simulink model "CLNN_sim_3dof_2NN"  (R2024b)
settings: Solver=ode1  StartTime=0.0  StopTime=T_all  FixedStep=T_sample  RelTol=1e-3
values from neighbouring files (symbols this model uses):
  a1 = m1 * lc1^2 + I1 + (m2 + m3) * l1^2    [plant_robot_3DoF_2NN.m]    (also in setting_3dof_2NN.m = 8.9995)
  a2 = I2 + m2 * lc2^2 + m3 * l2^2    [plant_robot_3DoF_2NN.m]    (also in setting_3dof_2NN.m = 8.9989)
  cl_tf = 300    [run_CLNN_3dof_2NN.m]
  cl_tf1 = 0    [run_CLNN_3dof_2NN.m]
  cl_tf2 = 1050    [run_CLNN_3dof_2NN.m]
  hidden_neure_count_q = 50    [run_CLNN_3dof_2NN.m]
  hidden_neure_count_s = 30    [run_CLNN_3dof_2NN.m]
  kq1 = 0.0026    [setting_3dof_2NN.m]
  kq2 = 0.0011    [setting_3dof_2NN.m]
  lamda = 5    [run_CLNN_3dof_2NN.m]
  lamda_cl = 0.2    [run_CLNN_3dof_2NN.m]
  lamda_cl_s = 0.2    [run_CLNN_3dof_2NN.m]
  learn_time = 100    [run_CLNN_3dof_2NN.m]
  M = [0.001 0 0 ... (first row only)    [run_CLNN_3dof_2NN.m]
  N = 3    [setting_3dof_2NN.m]
  noise_cov = 0    [setting_3dof_2NN.m]
  output_dimension_q = 1*N    [run_CLNN_3dof_2NN.m]
  output_dimension_s = 1*N    [run_CLNN_3dof_2NN.m]
  qd20 = 0    [run_CLNN_3dof_2NN.m]
  use_Tqr = 0    [run_CLNN_3dof_2NN.m]
(part 2 of 2)

== matlab function CLNN_sim_3dof_2NN/s/sd1 ==
  data: t input; q output; q2 output; dq2 output; dqq2 output; dqqq2 output; dqqqq2 output; learn_time input
function [q,q2,dq2,dqq2,dqqq2,dqqqq2]  = fcn(t, learn_time)

%% sim s1

a  = 0;  %paper pi / 12
w = 0;   %paper 2

a1 = 0.8 * pi / 1; %paper 0.8 * pi / 1
w1 = pi / 6;        % paper pi / 6  

if t> learn_time
    a1 = 0.8 * pi / 1; %paper 0.8 * pi / 1
    w1 = pi / 4;        % paper pi / 6  
end

q = 16 *( a1 * sin(w1 * t) + 1* 8 * pi);  %paper 1* 3 * pi


q2 = a * cos(w * t) - a + a1 * sin(w1 * t);
dq2 = -a * w * sin(w * t) + a1 * w1 * cos(w1 * t);
dqq2 = -a * w * w * cos(w * t) - a1 * w1 * w1 * sin(w1 * t);
dqqq2 = 0;
dqqqq2 = 0;
return;

== matlab function CLNN_sim_3dof_2NN/s/sd2 ==
  data: t input; q output; q2 output; dq2 output; dqq2 output; dqqq2 output; dqqqq2 output; learn_time input
function [q,q2,dq2,dqq2,dqqq2,dqqqq2]  = fcn(t, learn_time)
%% sim s2
a  = 0;  %paper pi / 12
w = 0;   %paper 2

a1 = 0.2 * pi / 1; % paper 0.2 * pi / 1; 
w1 = pi / 5;   % paper pi /5   

% if t > 80
%     w1 = pi / 8;
% elseif t > 50
%      w1 = pi / 7;
% elseif t > 20
%      w1 = pi / 6;
% end

if t> learn_time
    a1 = 0.2 * pi / 1; %paper 0.8 * pi / 1
    w1 = pi / 4;        % paper pi / 6  
end

q = 16 *( a1 * sin(w1 * t) + 1* 6 * pi);   % paper 1*3 * pi

q2 = a * cos(w * t) - a + a1 * sin(w1 * t) + pi/2;
dq2 = -a * w * sin(w * t) + a1 * w1 * cos(w1 * t);
dqq2 = -a * w * w * cos(w * t) - a1 * w1 * w1 * sin(w1 * t);
dqqq2 = 0;
dqqqq2 = 0;
return;

== matlab function CLNN_sim_3dof_2NN/s/sd3 ==
  data: t input; q output; q2 output; dq2 output; dqq2 output; dqqq2 output; dqqqq2 output; learn_time input
function [q,q2,dq2,dqq2,dqqq2,dqqqq2]  = fcn(t, learn_time)
%% sim s3
a  = 0;  %paper pi / 12
w = 0;   %paper 2
a1 = 0.2 * pi / 1; % paper 0.2 * pi / 1; 
w1 = pi / 5;   % paper pi /5   

if t> learn_time
    a1 = 0.2 * pi / 1; %paper 0.8 * pi / 1
    w1 = pi / 4;        % paper pi / 6  
end

q = 16 *( a1 * sin(w1 * t) + 1* 1* pi);   % paper 1*3 * pi

q2 = a * cos(w * t) - a + a1 * sin(w1 * t);
dq2 = -a * w * sin(w * t) + a1 * w1 * cos(w1 * t);
dqq2 = -a * w * w * cos(w * t) - a1 * w1 * w1 * sin(w1 * t);
dqqq2 = 0;
dqqqq2 = 0;
return;

== matlab function CLNN_sim_3dof_2NN/Theta_q/MATLAB Function Theta ==
  data: phi_filter_q input; phi_filter_phi_filter_q output; hidden_neure_count_q input
function phi_filter_phi_filter_q  = fcn(phi_filter_q,hidden_neure_count_q)
phi_filter_phi_filter_m = phi_filter_q * phi_filter_q';

phi_filter_phi_filter_q = phi_filter_phi_filter_m;
% phi_filter_phi_filter = zeros(625,625);

== matlab function CLNN_sim_3dof_2NN/THeta_WW_q/MATLAB Function Theta_W ==
  data: phi_filter_q input; phi_filter_W_q output; w_un_q_filter input; w_un_s_filter input
function phi_filter_W_q  = fcn(phi_filter_q,  w_un_q_filter, w_un_s_filter)
% w_un_filter = [w_un_q_filter; w_un_s_filter];
phi_filter_W_q = phi_filter_q * w_un_q_filter';

== matlab function CLNN_sim_3dof_2NN/THeta_WW_q/MATLAB Function ==
  data: u input; y output; t input; cl_tf1 input; cl_tf2 input
function y = fcn(u,t,cl_tf1, cl_tf2)
if t>cl_tf1 && t< cl_tf2
    y = u;
else
    y = zeros(51,3);  %41 x 6   (61,2)
end

== matlab function CLNN_sim_3dof_2NN/MATLAB Function6 ==
  data: output input; w_un_hat output; epsion output; w_norm_q output; w_norm_s output; controlu1 output; controlu2 output; u_theta1 output; u_theta2 output; pd_u output; model_u output; W_q output; hidden_neure_count_q input; hidden_neure_count_s input; N input; q input; W_s output
function [w_un_hat, epsion, w_norm_q,w_norm_s,controlu1, controlu2, u_theta1, u_theta2,pd_u, model_u, W_q, W_s] = fcn(output, hidden_neure_count_q,hidden_neure_count_s,N,q)
N = 3;
output_dimension = 2*N;

w_un_hat = output(1:output_dimension);
epsion =  output((output_dimension + 1):(2 * output_dimension));
controlu1 = output((2 * output_dimension +1):(2 * output_dimension + N));
controlu2 = output((2 * output_dimension + N +1):(2 * output_dimension + 2 * N));

pd_u = 0;
model_u = 0;
u_theta1 = q - controlu1;
u_theta2 = q - controlu2;


hidden_neure_count_q = 50; %40
hidden_neure_count_s = 30;
N_wq = N *(hidden_neure_count_q +1);
N_ws = N *(hidden_neure_count_s +1);

w_norm_temp_q = 0;
for i = (2 * output_dimension + 2 * N + 1):(N_wq + 2 * output_dimension + 2 * N)
    w_norm_temp_q = w_norm_temp_q + output(i) * output(i);
end
w_norm_q = w_norm_temp_q;

w_norm_temp_s = 0;
for i = (N_wq + 2 * output_dimension + 2 * N + 1):(N_wq + N_ws + 2 * output_dimension + 2 * N)
    w_norm_temp_s = w_norm_temp_s + output(i) * output(i);
end
w_norm_s = w_norm_temp_s;

W_q = output((2 * output_dimension + 2 * N + 1):(2 * output_dimension + 2 * N + N_wq));
W_s = output((2 * output_dimension + 2 * N + N_wq + 1):end);
